simulink model "plant"  (R2017b)
settings: Solver=VariableStepAuto  StartTime=0.0  StopTime=10.0  RelTol=1e-3
values from neighbouring files (symbols this model uses):
  m1 = 1    [project.m]
  m2 = 0.5    [project.m]
  theta = 50    [project.m]
undefined symbols (not defined in the file or in its folder): g, mu
libraries: simulink x1
settings Model: Creator=cassi  LastModifiedBy=cassi

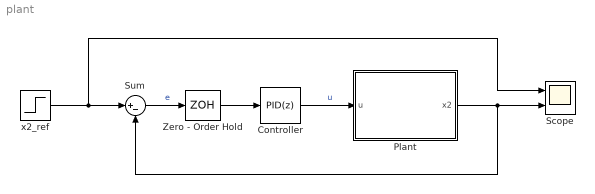
== system plant ==
  Controller : simulink/Continuous/PID Controller  Controller=PID  TimeDomain=Discrete-time  SampleTime=0.1  IntegratorMethod=Forward Euler  FilterMethod=Forward Euler  Form=Parallel  UseFilter=on  ControllerParametersSource=internal  P=0.0013736113613919  I=7.03007542263478e-06  D=0.0494584500254215  N=0.0820372386641655  InitialConditionSource=internal  InitialConditionForIntegrator=0  InitialConditionForFilter=0  ExternalReset=none  LimitOutput=off  UpperSaturationLimit=inf  LowerSaturationLimit=-inf  LinearizeAsGain=on  AntiWindupMode=none  Kb=1  TrackingMode=off  Kt=1  PParamMin=[]  PParamMax=[]  IParamMin=[]  IParamMax=[]  DParamMin=[]  DParamMax=[]  NParamMin=[]  NParamMax=[]  KbParamMin=[]  KbParamMax=[]  KtParamMin=[]  KtParamMax=[]  POutMin=[]  POutMax=[]  IOutMin=[]  IOutMax=[]  DOutMin=[]  DOutMax=[]  NOutMin=[]  NOutMax=[]  KbOutMin=[]  KbOutMax=[]  KtOutMin=[]  KtOutMax=[]  IntegratorOutMin=[]  IntegratorOutMax=[]  FilterOutMin=[]  FilterOutMax=[]  SumOutMin=[]  SumOutMax=[]  SumI1OutMin=[]  SumI1OutMax=[]  SumI2OutMin=[]  SumI2OutMax=[]  SumI3OutMin=[]  SumI3OutMax=[]  SumDOutMin=[]  SumDOutMax=[]  SaturationOutMin=[]  SaturationOutMax=[]  IntegratorContinuousStateAttributes=''  IntegratorStateMustResolveToSignalObject=off  IntegratorRTWStateStorageClass=Auto  FilterContinuousStateAttributes=''  FilterStateMustResolveToSignalObject=off  FilterRTWStateStorageClass=Auto  DifferentiatorICPrevScaledInput=0  DifferentiatorOutMin=[]  DifferentiatorOutMax=[]  InitialConditionSetting=State (most efficient)  FilterDiffOutCoefMin=[]  FilterDiffOutCoefMax=[]  SumDenOutMin=[]  SumDenOutMax=[]  SumNumOutMin=[]  SumNumOutMax=[]  ReciprocalOutMin=[]  ReciprocalOutMax=[]  DivideOutMin=[]  DivideOutMax=[]  TunerSelectOption=Transfer Function Based (PID Tuner App)
  Plant : Subsystem
  Scope : Scope  NumInputPorts=2
  Sum : Sum  Inputs=|+-
  Zero - Order Hold : ZeroOrderHold  SampleTime=0.1
  x2_ref : Step  After=10  SampleTime=0
  wires:
  Controller/1 -> Plant/1(u)  "u"
  Plant/1(x2) -> Sum/2, Scope/2
  x2_ref/1 -> Scope/1, Sum/1
  Sum/1 -> Zero - Order Hold/1  "e"
  Zero - Order Hold/1 -> Controller/1

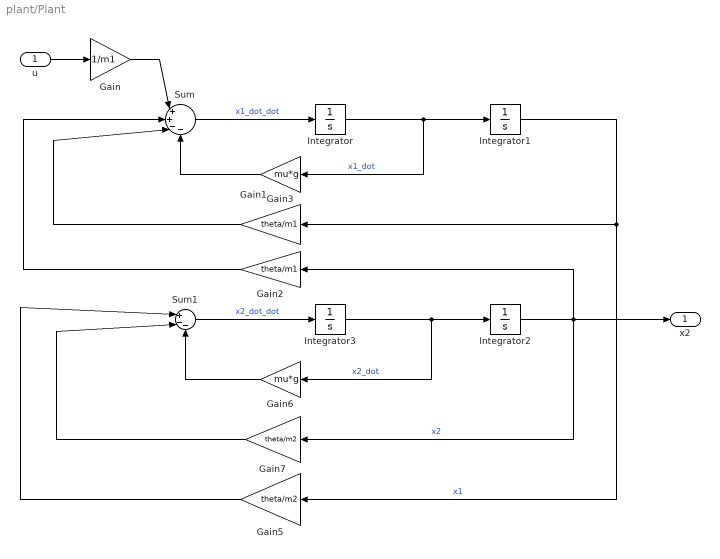
== system plant/Plant ==
  u : Inport  SampleTime=0.1
  Gain : Gain  Gain=1/m1
  Gain1 : Gain  Gain=theta/m1
  Gain2 : Gain  Gain=theta/m1
  Gain3 : Gain  Gain=mu*g
  Gain5 : Gain  Gain=theta/m2
  Gain6 : Gain  Gain=mu*g
  Gain7 : Gain  Gain=theta/m2
  Integrator{,1..3} (4 alike) : Integrator
  Sum : Sum  Inputs=|++--
  Sum1 : Sum  Inputs=|+--
  x2 : Outport
  wires:
  Integrator3/1 -> Integrator2/1, Gain6/1  "x2_dot"
  Integrator/1 -> Integrator1/1, Gain3/1  "x1_dot"
  Sum/1 -> Integrator/1  "x1_dot_dot"
  Integrator1/1 -> Gain5/1, Gain1/1  "x1"
  Gain7/1 -> Sum1/2
  Gain2/1 -> Sum/2
  Gain3/1 -> Sum/4
  Gain6/1 -> Sum1/3
  Sum1/1 -> Integrator3/1  "x2_dot_dot"
  Gain5/1 -> Sum1/1
  Integrator2/1 -> x2/1, Gain2/1, Gain7/1  "x2"
  Gain1/1 -> Sum/3
  u/1 -> Gain/1
  Gain/1 -> Sum/1
